simulink model "wesrf_cartesian_pose_motion"  (R2020b)
settings: Solver=FixedStepDiscrete  StartTime=0.0  StopTime=inf  FixedStep=0.001  RelTol=1e-3  EnableMultiTasking=on
PreLoadFcn:
  | demos_common_configs();
undefined symbols (not defined in the file or in its folder): DiscIntNeverNeededParam
libraries: franka_simulink_library x9, simulink x2, franka_simulink_library_misc x2, robotcorelib x1
settings Model: SimulationMode=external  ExtModeTrigDuration=50000  ExtModeArchiveMode=auto  ExtModeArchiveFileName=data  ExtModeArchiveDirName=/home/host/franka_matlab_v0.2.0/WESRF_workingDir/data/output_data/pose_motion_tracking  ExtModeAddSuffixToVar=on  Creator=vasi_ko  LastModifiedBy=root
settings DataIOCC: LimitDataPoints=on  SaveFormat=Array  ReturnWorkspaceOutputs=off
settings OptimizationCC: DefaultParameterBehavior=Inlined  EnhancedBackFolding=on  PassReuseOutputArgsAs=Individual arguments  ZeroExternalMemoryAtStartup=off  ZeroInternalMemoryAtStartup=off  OptimizeBlockOrder=speed  DifferentSizesBufferReuse=on  OptimizationCustomize=off  EfficientTunableParamExpr=on
settings DebuggingCC: SolverPrmCheckMsg=warning  ParameterTunabilityLossMsg=error  SFUnexpectedBacktrackingDiag=warning  SFNoUnconditionalDefaultTransitionDiag=warning  SFExecutionAtInitializationDiag=none  ArithmeticOperatorsInVariantConditions=warning
settings HardwareCC: ProdBitPerLong=64  ProdHWDeviceType=Intel->x86-64 (Linux 64)
settings ModelReferenceCC: PropagateSignalLabelsOutOfModel=off
settings SFSimCC: SimUseLocalCustomCode=off  MATLABDynamicMemAlloc=off  CustomCodeUndefinedFunction=UseInterfaceOnly  SimTargetLang=C++
settings RTWCC: Description=Embedded Coder  SystemTargetFile=franka_emika_panda.tlc  GenCodeOnly=on  TemplateMakefile=ert_default_tmf  RTWVerbose=off  RTWUseLocalCustomCode=off  Toolchain=Franka Simulink | gmake (64-bit linux)  BuildConfiguration=Faster Runs  TargetLang=C++
settings CodeAppCC: ForceParamTrailComments=on  IgnoreCustomStorageClasses=off  OperatorAnnotations=on  SimulinkDataObjDesc=on  SFDataObjDesc=on  InsertBlockDesc=on
settings STFCustomTargetCC: TargetLangStandard=C99 (ISO)  MultiwordLength=256  GenerateSampleERTMain=on  ModelReferenceCompliant=off  ConcurrentExecutionCompliant=off  CombineOutputUpdateFcns=on  ERTCustomFileBanners=on  SupportNonInlinedSFcns=off  RemoveResetFunc=on  MATLABClassNameForMDSCustomization=Simulink.SoftwareTarget.ERTCustomization  GRTInterface=off  UseToolchainInfoCompliant=on  SystemTargetFile=franka_emika_panda.tlc
settings ERTTargetCC: TargetLangStandard=C99 (ISO)  GenerateSampleERTMain=on  ModelReferenceCompliant=off  ParMdlRefBuildCompliant=off  CompOptLevelCompliant=off  ConcurrentExecutionCompliant=off  SupportContinuousTime=on  ModelStepFunctionPrototypeControlCompliant=off  ExtMode=on  ExtModeMexArgs='172.16.0.1' 0 17725  InlinedParameterPlacement=NonHierarchical  ERTCustomFileTemplate=franka_emika_panda_file_process.tlc
settings ConfigComp: CovMetricSettings=dw  CovSaveCumulativeToWorkspaceVar=on  CovSaveSingleToWorkspaceVar=on  CovExternalEMLEnable=off  CovSFcnEnable=off

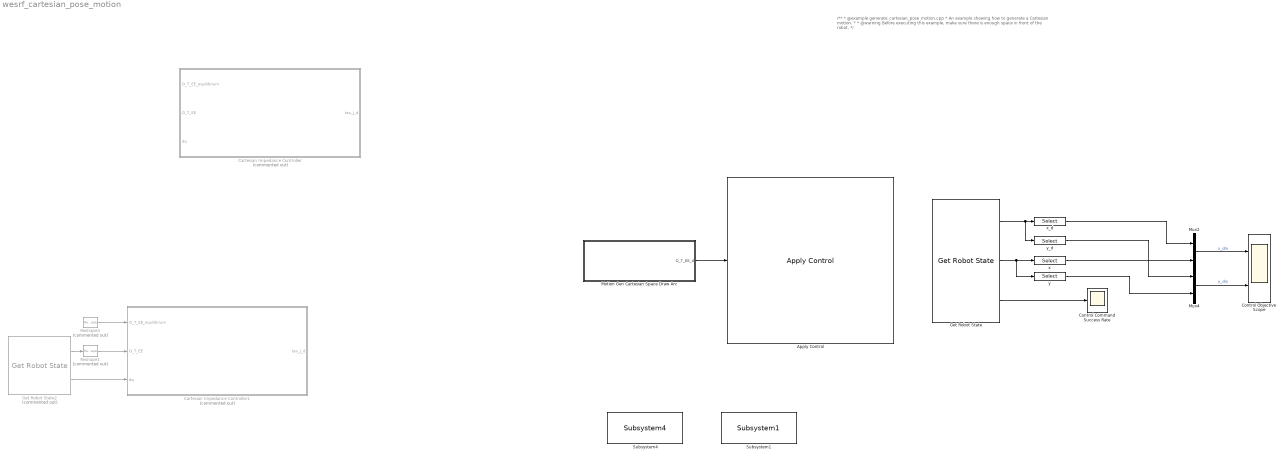
== system wesrf_cartesian_pose_motion ==
  note: /**
      |  * @example generate_cartesian_pose_motion.cpp
      |  * An example showing how to generate a Cartesian motion.
      |  *
      |  * @warning Before executing this example, make sure there is enough space in front of the robot.
      |  */
  Apply Control : franka_simulink_library/Apply Control  robot_ip=robot_ip  gripper_attached=off  control_mode=Cartesian Pose - Internal Controller Mode  controller_choice=Joint Impedance Controller  elbow_control=off  collision_thresholds=[25.0, 25.0, 22.0, 20.0, 19.0, 17.0, 14.0,35.0, 35.0, 32.0, 30.0, 29.0, 27.0, 24.0,25.0, 25.0, 22.0, 20.0, 19.0, 17.0, 14.0,35.0, 35.0, 32.0, 30.0, 29.0, 27.0, 24.0,30.0, 30.0, 30.0, 25.0, 25.0, 25.0,40.0, 40.0, 40.0, 35.0, 35.0, 35.0,30.0, 30.0, 30.0, 25.0, 25.0, 25.0,40.0, 40.0, 40.0, 35.0, 35.0, 35.0]  joint_impedance=[3000, 3000, 3000, 2500, 2500, 2000, 2000]  cartesian_impedance=cartesian_impedance  load_inertia=load_inertia  EE_T_K=EE_T_K  init_joint_configuration_req=on  init_joint_configuration=q_init
      settings: SourceProductName=Franka Emika
  Cartesian Impedance Controller : Subsystem  Commented=on
      mask Display:
      | disp('{\bf\fontsize{18}Cartesian Impedance Controller}', 'texmode','on');
      | 
      | block_icon('Controller')
      | 
      | port_label('output',1,'tau_J_d');
      | 
      | port_label('input',1,'O_T_EE_equilibrium');
      | port_label('input',2,'O_T_EE');
      | port_label('input',3,'dq');
  Cartesian Impedance Controller1 : Subsystem  Commented=on
      mask Display:
      | disp('{\bf\fontsize{18}Cartesian Impedance Controller}', 'texmode','on');
      | 
      | block_icon('Controller')
      | 
      | port_label('output',1,'tau_J_d');
      | 
      | port_label('input',1,'O_T_EE_equilibrium');
      | port_label('input',2,'O_T_EE');
      | port_label('input',3,'dq');
  Control Command Success Rate : Scope
  Control Objective Scope : Scope  NumInputPorts=2
  Get Robot State : franka_simulink_library/Get Robot State  robot_ip=robot_ip  signals_requested='O_T_EE_d O_T_EE control_command_success_rate'
      settings: SourceProductName=Franka Emika
  Get Robot State2 : franka_simulink_library/Get Robot State  Commented=on  robot_ip=robot_ip  signals_requested='O_T_EE dq'
      settings: SourceProductName=Franka Emika
  Motion Gen Cartesian Space Draw Arc : Subsystem
      mask Display:
      | pos = get_param(gcb, 'Position');
      | width = pos(3) - pos(1);
      | x = [0:width];
      | y = sin(x/180*pi);
      | % Parameters 'm' and 'b' must be defined in 'Parameters & Dialog' pane.
      | plot(cos(x/180*pi*0.5), sin(x/180*pi*0.5));
      | 
      | port_label('output',1,'O_T_EE_d');
  Mux2 : Mux  Inputs=2
  Mux4 : Mux  Inputs=2
  Reshape1 : Reshape  Commented=on  OutputDimensionality=Customize  OutputDimensions=[4,4]
  Reshape3 : Reshape  Commented=on  OutputDimensionality=Customize  OutputDimensions=[4,4]
  Subsystem1 : franka_simulink_library_misc/Subsystem1  SystemSampleTime=-1  VariantActivationTime=update diagram  Latency=0  AutoFrameSizeCalculation=off
  Subsystem4 : franka_simulink_library_misc/Subsystem4  SystemSampleTime=-1  VariantActivationTime=update diagram  Latency=0  AutoFrameSizeCalculation=off
  x : Selector  InputPortWidth=16  IndexOptions=Index vector (dialog)  Indices=13  OutputSizes=1
  x_d : Selector  InputPortWidth=16  IndexOptions=Index vector (dialog)  Indices=13  OutputSizes=1
  y : Selector  InputPortWidth=16  IndexOptions=Index vector (dialog)  Indices=14  OutputSizes=1
  y_d : Selector  InputPortWidth=16  IndexOptions=Index vector (dialog)  Indices=14  OutputSizes=1
  wires:
  x/1 -> Mux2/2
  y/1 -> Mux4/2
  Mux2/1 -> Control Objective Scope/1  "x_d/x"
  Get Robot State/1 -> y_d/1, x_d/1
  x_d/1 -> Mux2/1
  y_d/1 -> Mux4/1
  Get Robot State/2 -> y/1, x/1
  Get Robot State/3 -> Control Command Success Rate/1
  Mux4/1 -> Control Objective Scope/2  "y_d/y"
  Reshape1/1 -> Cartesian Impedance Controller1/2(O_T_EE)
  Get Robot State2/2 -> Cartesian Impedance Controller1/3(dq)
  Reshape3/1 -> Cartesian Impedance Controller1/1(O_T_EE_equilibrium)
  Get Robot State2/1 -> Reshape1/1
  Motion Gen Cartesian Space Draw Arc/1(O_T_EE_d) -> Apply Control/1

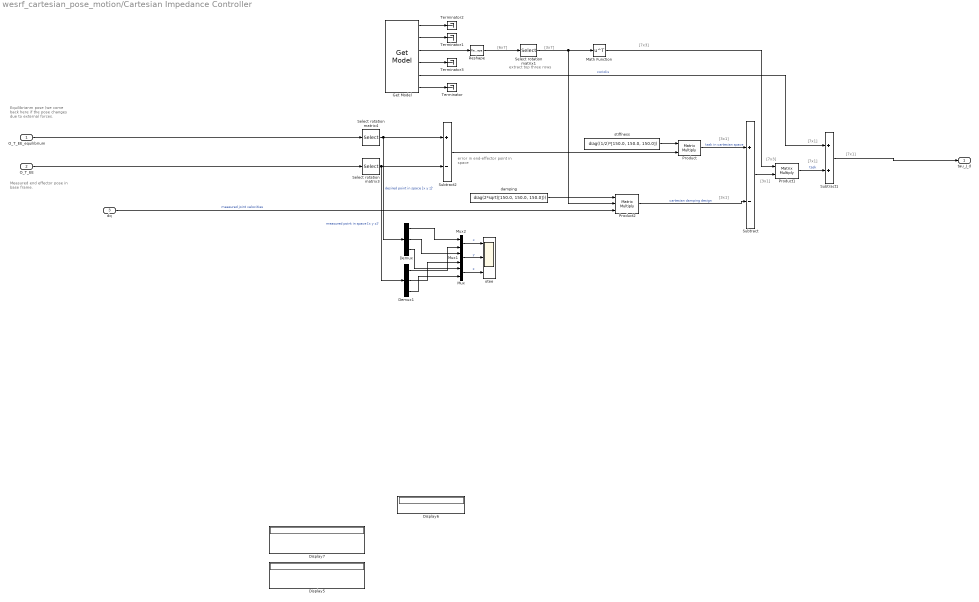
== system wesrf_cartesian_pose_motion/Cartesian Impedance Controller ==
  note: extract top three rows
  note: [7x1]
  note: [3x1]
  note: [7x3]
  note: [3x7]
  note: [6x7]
  note: Measured end effector pose in base frame.
  note: error in end-effector point in space
  note: Equilibrianm pose (we come back here if the pose changes due to external forces.
  note: [3x1]
  note: [3x1]
  note: [7x3]
  note: [7x1]
  note: [7x1]
  O_T_EE_equilibrium : Inport
  O_T_EE : Inport  Port=2
  dq : Inport  Port=3
  Demux : Demux  Outputs=3
  Demux1 : Demux  Outputs=3
  Display5 : Display
  Display6 : Display
  Display7 : Display
  Get Model : franka_simulink_library/Get Model  robot_ip=robot_ip
      settings: SourceProductName=Franka Emika
  Math Function : Math  Operator=transpose  SignedPower=on  SaturateOnIntegerOverflow=on
  Mux : Mux  Inputs=2
  Mux1 : Mux  Inputs=2
  Mux2 : Mux  Inputs=2
  Product : Product  Multiplication=Matrix(*)
  Product1 : Product  Multiplication=Matrix(*)
  Product2 : Product  Inputs=3  Multiplication=Matrix(*)
  Reshape : Reshape  OutputDimensionality=Customize  OutputDimensions=[6,7]
  Select rotation matrix1 : Selector  NumberOfDimensions=2  InputPortWidth=3  IndexOptions=Index vector (dialog),Index vector (dialog)  Indices=[1,2,3],[1 2 3 4 5 6 7]  OutputSizes=1
  Select rotation matrix3 : Selector  NumberOfDimensions=2  InputPortWidth=3  IndexOptions=Index vector (dialog),Index vector (dialog)  Indices=[1,2,3],[4]  OutputSizes=1
  Select rotation matrix4 : Selector  NumberOfDimensions=2  InputPortWidth=3  IndexOptions=Index vector (dialog),Index vector (dialog)  Indices=[1,2,3],[4]  OutputSizes=1
  Subtract : Sum  Inputs=+-
  Subtract1 : Sum
  Subtract2 : Sum  Inputs=+-
  Terminator{,1..3} (4 alike) : Terminator
  damping : Constant  Value=diag(2*sqrt([150.0, 150.0, 150.0]))  VectorParams1D=off
  otee : Scope  NumInputPorts=3
  stiffness : Constant  Value=diag((1/2)*[150.0, 150.0, 150.0])  VectorParams1D=off
  tau_J_d : Outport  VectorParamsAs1DForOutWhenUnconnected=off
  wires:
  Get Model/6 -> Terminator/1
  Get Model/2 -> Terminator1/1
  Get Model/1 -> Terminator2/1
  Get Model/4 -> Terminator3/1
  stiffness/1 -> Product/1
  Math Function/1 -> Product1/1
  Product/1 -> Subtract/1  "task in cartesian space"
  Product2/1 -> Subtract/2  "cartesian damping design"
  Get Model/5 -> Subtract1/1  "coriolis"
  dq/1 -> Product2/3  "measured joint velocities"
  damping/1 -> Product2/1
  Subtract1/1 -> tau_J_d/1
  Product1/1 -> Subtract1/2  "task"
  O_T_EE/1 -> Select rotation matrix3/1
  O_T_EE_equilibrium/1 -> Select rotation matrix4/1
  Select rotation matrix4/1 -> Demux/1, Subtract2/1  "desired point in space [x y z]'"
  Select rotation matrix3/1 -> Demux1/1, Subtract2/2  "measured point in space [x y z]'"
  Subtract/1 -> Product1/2
  Subtract2/1 -> Product/2
  Select rotation matrix1/1 -> Math Function/1, Product2/2
  Reshape/1 -> Select rotation matrix1/1
  Get Model/3 -> Reshape/1
  Demux/1 -> Mux2/1
  Demux1/1 -> Mux2/2
  Demux/2 -> Mux1/1
  Demux1/2 -> Mux1/2
  Demux/3 -> Mux/1
  Demux1/3 -> Mux/2
  Mux1/1 -> otee/2  "y"
  Mux2/1 -> otee/1  "x"
  Mux/1 -> otee/3  "z"

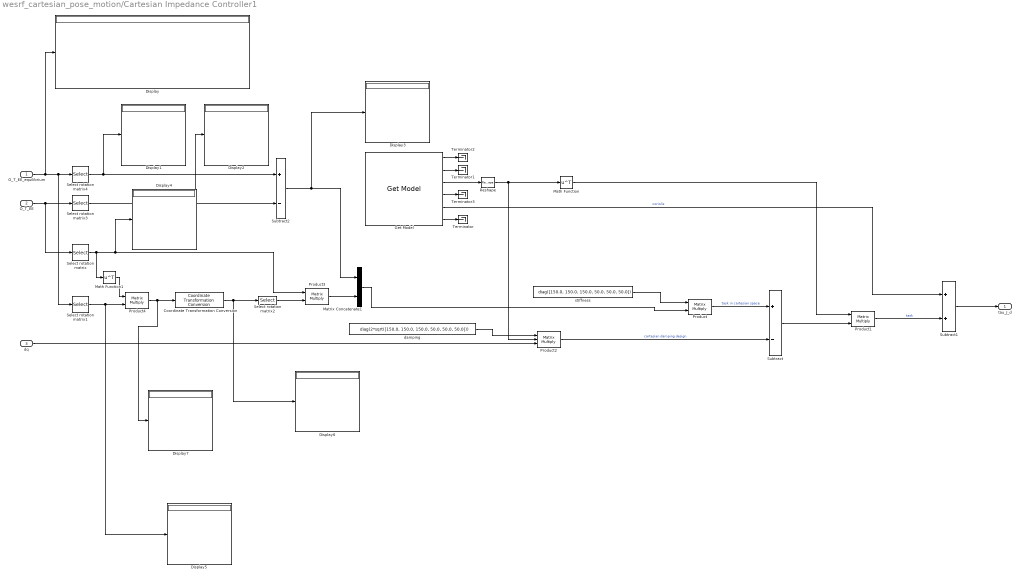
== system wesrf_cartesian_pose_motion/Cartesian Impedance Controller1 ==
  O_T_EE_equilibrium : Inport
  O_T_EE : Inport  Port=2
  dq : Inport  Port=3
  Coordinate Transformation Conversion : robotcorelib/Coordinate Transformation Conversion  InputRepresentation=Rotation Matrix  InputEulerSequence=ZYX  ShowTrVecInputPort=on  OutputRepresentation=Quaternion  OutputEulerSequence=ZYX  ShowTrVecOutputPort=on  SimulateUsing=Code generation
      settings: SourceProductBaseCode=NV,RO,RR,UV
  Display{,1..7} (8 alike) : Display
  Get Model : franka_simulink_library/Get Model  robot_ip=robot_ip
      settings: SourceProductName=Franka Emika
  Math Function : Math  Operator=transpose  SignedPower=on  SaturateOnIntegerOverflow=on
  Math Function1 : Math  Operator=transpose  SignedPower=on  SaturateOnIntegerOverflow=on
  Matrix Concatenate1 : Concatenate
  Product{,1,3..4} (4 alike) : Product  Multiplication=Matrix(*)
  Product2 : Product  Inputs=3  Multiplication=Matrix(*)
  Reshape : Reshape  OutputDimensionality=Customize  OutputDimensions=[6,7]
  Select rotation matrix : Selector  NumberOfDimensions=2  InputPortWidth=3  IndexOptions=Index vector (dialog),Index vector (dialog)  Indices=[1,2,3],[1 2 3]  OutputSizes=1
  Select rotation matrix1 : Selector  NumberOfDimensions=2  InputPortWidth=3  IndexOptions=Index vector (dialog),Index vector (dialog)  Indices=[1,2,3],[1 2 3]  OutputSizes=1
  Select rotation matrix2 : Selector  InputPortWidth=4  IndexOptions=Index vector (dialog)  Indices=[2,3,4]  OutputSizes=1
  Select rotation matrix3 : Selector  NumberOfDimensions=2  InputPortWidth=3  IndexOptions=Index vector (dialog),Index vector (dialog)  Indices=[1,2,3],[4]  OutputSizes=1
  Select rotation matrix4 : Selector  NumberOfDimensions=2  InputPortWidth=3  IndexOptions=Index vector (dialog),Index vector (dialog)  Indices=[1,2,3],[4]  OutputSizes=1
  Subtract : Sum  Inputs=+-
  Subtract1 : Sum
  Subtract2 : Sum  Inputs=+-
  Terminator{,1..3} (4 alike) : Terminator
  damping : Constant  Value=diag(2*sqrt([150.0, 150.0, 150.0, 50.0, 50.0, 50.0]))  VectorParams1D=off
  stiffness : Constant  Value=diag([150.0, 150.0, 150.0, 50.0, 50.0, 50.0])  VectorParams1D=off
  tau_J_d : Outport  VectorParamsAs1DForOutWhenUnconnected=off
  wires:
  Get Model/6 -> Terminator/1
  Get Model/2 -> Terminator1/1
  Get Model/1 -> Terminator2/1
  Get Model/4 -> Terminator3/1
  Get Model/3 -> Reshape/1
  Reshape/1 -> Product2/2, Math Function/1
  stiffness/1 -> Product/1
  Math Function/1 -> Product1/1
  Product/1 -> Subtract/1  "task in cartesian space"
  Product2/1 -> Subtract/2  "cartesian damping design"
  Get Model/5 -> Subtract1/1  "coriolis"
  dq/1 -> Product2/3
  damping/1 -> Product2/1
  Subtract1/1 -> tau_J_d/1
  Product1/1 -> Subtract1/2  "task"
  O_T_EE/1 -> Select rotation matrix3/1, Select rotation matrix/1
  O_T_EE_equilibrium/1 -> Display/1, Select rotation matrix4/1, Select rotation matrix1/1
  Select rotation matrix4/1 -> Display1/1, Subtract2/1
  Select rotation matrix3/1 -> Subtract2/2, Display2/1
  Subtract2/1 -> Display3/1, Matrix Concatenate1/1
  Coordinate Transformation Conversion/1 -> Display6/1, Select rotation matrix2/1
  Product4/1 -> Display7/1, Coordinate Transformation Conversion/1
  Subtract/1 -> Product1/2
  Select rotation matrix2/1 -> Product3/2
  Matrix Concatenate1/1 -> Product/2
  Select rotation matrix/1 -> Math Function1/1, Display4/1, Product3/1
  Product3/1 -> Matrix Concatenate1/2
  Select rotation matrix1/1 -> Display5/1, Product4/2
  Math Function1/1 -> Product4/1

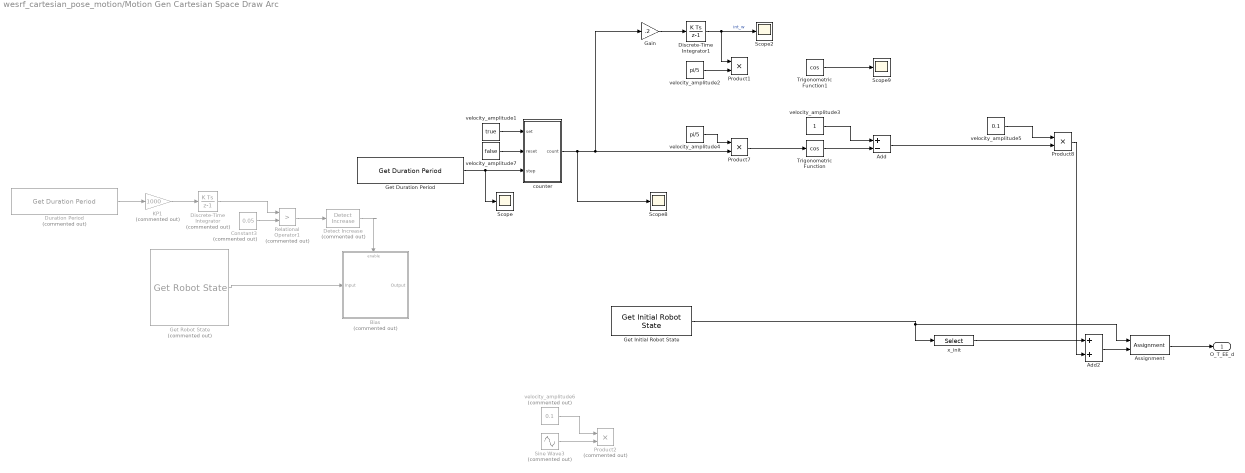
== system wesrf_cartesian_pose_motion/Motion Gen Cartesian Space Draw Arc ==
  Add : Sum  Inputs=+-
  Add2 : Sum
  Assignment : Assignment  DiagnosticForDimensions=Warning  IndexOptions=Index vector (dialog)  Indices=13  OutputSizes=1
  Bias : Subsystem  Commented=on
  Constant3 : Constant  Commented=on  Value=0.05
  Detect Increase : simulink/Logic and Bit Operations/Detect Increase  Commented=on  vinit=0.0  OutDataTypeStr=boolean
  Discrete-Time Integrator : DiscreteIntegrator  Commented=on  SampleTime=-1  ICPrevOutput=DiscIntNeverNeededParam  ICPrevScaledInput=DiscIntNeverNeededParam
  Discrete-Time Integrator1 : DiscreteIntegrator  SampleTime=1e-3  ICPrevOutput=DiscIntNeverNeededParam  ICPrevScaledInput=DiscIntNeverNeededParam
  Duration Period : franka_simulink_library/Get Duration Period  Commented=on  robot_ip=robot_ip
      settings: SourceProductName=Franka Emika
  Gain : Gain  Gain=.2
  Get Duration Period : franka_simulink_library/Get Duration Period  robot_ip=robot_ip
      settings: SourceProductName=Franka Emika
  Get Initial Robot State : franka_simulink_library/Get Initial Robot State  robot_ip=robot_ip  signals_requested='O_T_EE'
      settings: SourceProductName=Franka Emika
  Get Robot State : franka_simulink_library/Get Robot State  Commented=on  robot_ip=robot_ip  signals_requested='O_T_EE'
      settings: SourceProductName=Franka Emika
  KP1 : Gain  Commented=on  Gain=1000
  Product1 : Product
  Product2 : Product  Commented=on
  Product7 : Product
  Product8 : Product
  Relational Operator1 : RelationalOperator  Commented=on  Operator=>  OutDataTypeStr=boolean  RndMeth=Nearest
  Scope{,2,8..9} (4 alike) : Scope
  Sine Wave3 : Sin  Commented=on  SineType=Sample based  Bias=1  Samples=10e3  SampleTime=1e-3  Offset=7500
  Trigonometric Function : Trigonometry  Operator=cos  NumberOfIterations=50
  Trigonometric Function1 : Trigonometry  Operator=cos  NumberOfIterations=50
  counter : Subsystem
  velocity_amplitude1 : Constant  Value=true  VectorParams1D=off
  velocity_amplitude2 : Constant  Value=pi/5  VectorParams1D=off
  velocity_amplitude3 : Constant  VectorParams1D=off
  velocity_amplitude4 : Constant  Value=pi/5  VectorParams1D=off
  velocity_amplitude5 : Constant  Value=0.1  VectorParams1D=off
  velocity_amplitude6 : Constant  Commented=on  Value=0.1  VectorParams1D=off
  velocity_amplitude7 : Constant  Value=false  VectorParams1D=off
  x_init : Selector  InputPortWidth=16  IndexOptions=Index vector (dialog)  Indices=13  OutputSizes=1
  O_T_EE_d : Outport  VectorParamsAs1DForOutWhenUnconnected=off
  wires:
  Duration Period/1 -> KP1/1
  KP1/1 -> Discrete-Time Integrator/1
  Relational Operator1/1 -> Detect Increase/1
  Discrete-Time Integrator/1 -> Relational Operator1/1
  Constant3/1 -> Relational Operator1/2
  Detect Increase/1 -> Bias/Enable
  Get Robot State/1 -> Bias/1(Input)
  Discrete-Time Integrator1/1 -> Product1/1, Scope2/1  "int_w"
  Gain/1 -> Discrete-Time Integrator1/1
  Get Initial Robot State/1 -> Assignment/1, x_init/1
  Add2/1 -> Assignment/2
  Get Duration Period/1 -> Scope/1, counter/3(step)
  velocity_amplitude7/1 -> counter/2(reset)
  velocity_amplitude1/1 -> counter/1(set)
  velocity_amplitude3/1 -> Add/1
  velocity_amplitude5/1 -> Product8/1
  counter/1(count) -> Scope8/1, Product7/2, Gain/1
  velocity_amplitude2/1 -> Product1/2
  Trigonometric Function1/1 -> Scope9/1
  velocity_amplitude4/1 -> Product7/1
  Product7/1 -> Trigonometric Function/1
  Trigonometric Function/1 -> Add/2
  Add/1 -> Product8/2
  velocity_amplitude6/1 -> Product2/1
  Sine Wave3/1 -> Product2/2
  x_init/1 -> Add2/1
  Assignment/1 -> O_T_EE_d/1
  Product8/1 -> Add2/2

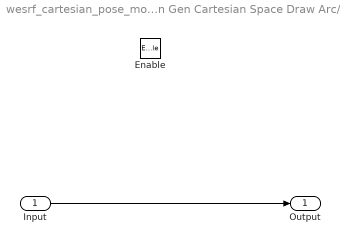
== system wesrf_cartesian_pose_motion/Motion Gen Cartesian Space Draw Arc/Bias ==
  Input : Inport
  Enable : EnablePort
  Output : Outport
  wires:
  Input/1 -> Output/1

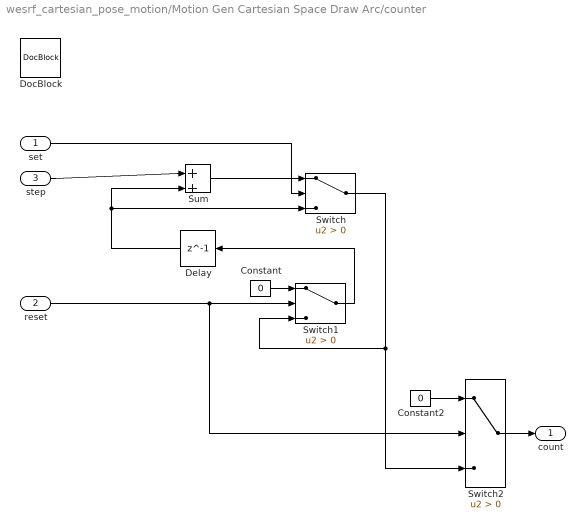
== system wesrf_cartesian_pose_motion/Motion Gen Cartesian Space Draw Arc/counter ==
  set : Inport  OutDataTypeStr=boolean
  reset : Inport  Port=2  OutDataTypeStr=boolean
  step : Inport  Port=3  OutDataTypeStr=double
  Constant : Constant  Value=0  OutDataTypeStr=double
  Constant2 : Constant  Value=0  OutDataTypeStr=double
  Delay : Delay  DelayLength=1  InitialCondition=0
  DocBlock : simulink/Model-Wide Utilities/DocBlock  DocumentType=Text
      content=|
      | %% counter
      | %
      | % This library includes the counter functionality that increases
      | % it's output by an input step factor for each computational step. The counter
      | % can also be externaly reset.
      | % -----------------------------------------------------------------------
      | % Author    : Konstantinos Vasios
      | % Date      : 01.09.2017
      | % Copyright : Franka Emika GmbH
      | % -----------------------------------------------------------------------
      | %
      | % Inputs:
      | % @param set : activates the counter. (data type: boolean, dimension: 1)
      | % @param reset: it resets the counter. Count starts from 0. (data type: boolean, dimension: 1)
      | % @param step: increment factor. (data type: real, dimension: 1)
      | %
      | % Outputs:
      | % @return count: current counter value. (data type: real, dimension: 1)
      | %% -----------------------------------------------------------------------
  Sum : Sum  Inputs=|++
  Switch : Switch  Criteria=u2 > Threshold
  Switch1 : Switch  Criteria=u2 > Threshold  OutDataTypeStr=double
  Switch2 : Switch  Criteria=u2 > Threshold  OutDataTypeStr=double
  count : Outport  OutDataTypeStr=double  VectorParamsAs1DForOutWhenUnconnected=off
  wires:
  Switch1/1 -> Delay/1
  Constant/1 -> Switch1/1
  reset/1 -> Switch2/2, Switch1/2
  Delay/1 -> Switch/3, Sum/2
  step/1 -> Sum/1
  Switch/1 -> Switch2/3, Switch1/3
  set/1 -> Switch/2
  Sum/1 -> Switch/1
  Constant2/1 -> Switch2/1
  Switch2/1 -> count/1
